simulink model "HESS_VBWF"  (R2023a)
settings: Solver=FixedStepAuto  StartTime=0.0  StopTime=2.5  RelTol=1e-3
undefined symbols (not defined in the file): Acid, BE, Lead, ode23tb, trap, Ts
libraries: spsMosfetLib x5, spsSeriesRLCBranchLib x5, slpidlib x3, spsCurrentMeasurementLib x3, spsPWMGeneratorDCDCLib x2, spsMeanLib x2, rfmathmodels2 x1, spsBatteryLib x1, spsVoltageMeasurementLib x1, spsPVArrayLib x1, spsDiodeLib x1, spsSupercapacitorLib x1
settings Model: Creator=bomma  LastModifiedBy=bomma

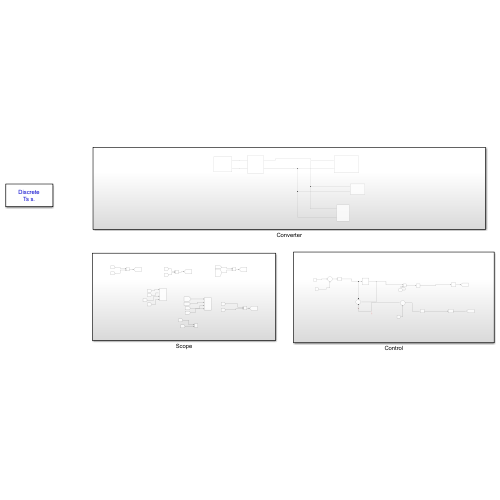
[thumbnail: Simulink's stored preview of the top-level diagram]
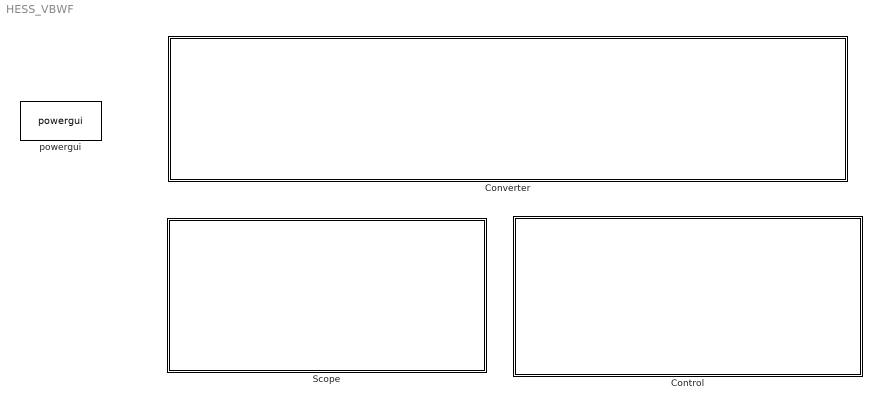
== system HESS_VBWF ==
  Control : Subsystem
  Converter : Subsystem
  Scope : Subsystem
  powergui : spspowerguiLib/powergui  Priority=1  SimulationMode=Discrete  SampleTime=Ts  frequency=60  Iterations=50  frequencyindice=0  Pbase=100e6  ErrMax=1e-4  UnitsV=kV  UnitsW=MW  buscounter=0  FunctionMessages=off  echomessages=off  EnableUseOfTLC=off  CurrentSourceSwitches=off  DisableSnubberDevices=off  DisableRonSwitches=off  DisableVfSwitches=off  DisplayEquations=off  AutomaticDiscreteSolvers=off  SolverType=Tustin/Backward Euler (TBE)  Interpol=off  ExternalGateDelay=off  methode=off  Ts=100  x0status=blocks  SPID=on  SwTol=0  HookPort=off  NonlinearTolerance=1e-4  nMaxIteration=100  ContinueOnMaxIteration=off  RestoreLinks=warning  ResistiveCurrentMeasurement=off  Frange=[0:2:500]  Ylog=off  Xlog=on  ShowGrid=off  save=off  variable=ZData  structure=0  ZoomFFT=off  StartTime=0.0  cycles=1  DisplayStyle=1  fundamental=60  FreqAxis=off  MaxFrequency=1000  frequencyindicesteady=1  RmsSteady=1  display=off

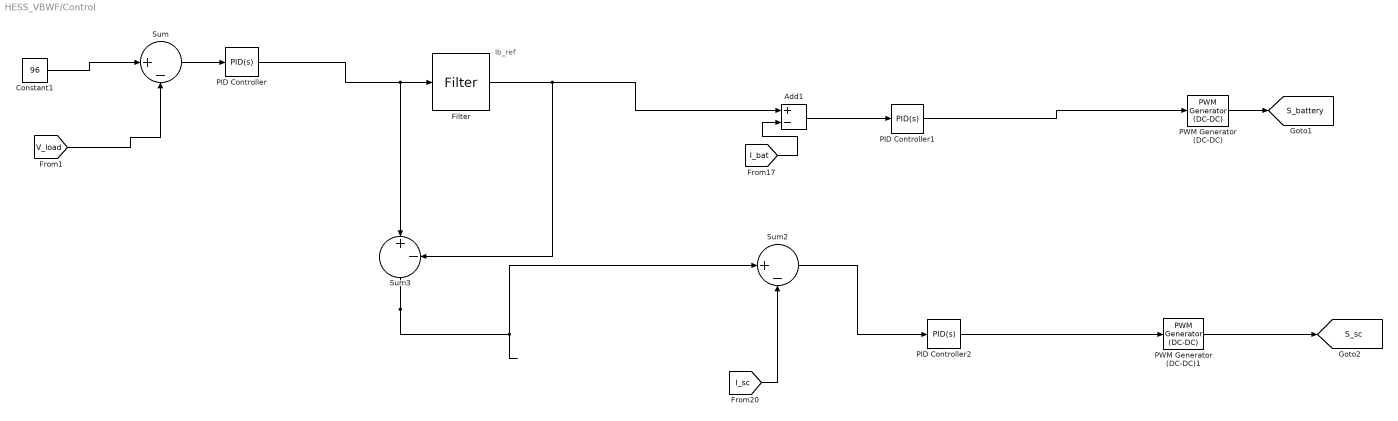
== system HESS_VBWF/Control ==
  note: Ib_ref
  Add1 : Sum  Inputs=+-
  Constant1 : Constant  Value=96
  Filter : rfmathmodels2/Filter  DesignMethod=Butterworth  ResponseType=Lowpass  UseFilterOrder=on  FilterOrder=3  PassFreq_lp=1e9  PassFreq_hp=2000000000  PassFreq_bp=[2000000000 3000000000]  PassFreq_bs=[1000000000 4000000000]  PassAtten=10*log10(2)  StopFreq_lp=2000000000  StopFreq_hp=1000000000  StopFreq_bp=[1500000000 3500000000]  StopFreq_bs=[2100000000 2900000000]  StopAtten=40  CarrierFrequency=1e9  SignalBandwidth=10000000  SimulateUsing=Interpreted execution  ModelingDomain=Time domain (Fixed step)  SolverFixedStep=NDF2  SolverODE=ode23tb (trap+BE)  PoleFitting=Share all poles  RationalArguments={ 'Tolerance', -40, 'TendsToZero', false, 'MaxPoles', 48, 'Qlimit', inf }  LengthFIR=128  PlotType1=S21  Plot1Units=Magnitude (dB)  Plot1ArgumentsImpulse=[1e-11 1e4]  Plot1ArgumentsStep=[1e-11 1e4 1e-10]  PlotType2=None  Plot2Units=Magnitude (dB)  Plot2ArgumentsImpulse=[1e-11 1e4]  Plot2ArgumentsStep=[1e-11 1e4 1e-10]  FrequencyPoints=logspace(8,10,2001)  XaxisScale=Linear  YaxisScale=Linear
  PID Controller : slpidlib/PID Controller  Controller=PID  Form=Parallel  TimeDomain=Continuous-time  UseExternalTs=off  SampleTime=-1  IntegratorMethod=Forward Euler  FilterMethod=Forward Euler  ControllerParametersSource=internal  P=1  I=1  UseKiTs=off  D=0  N=100  UseFilter=on  TunerSelectOption=Transfer Function Based (PID Tuner App)  InitialConditionSource=internal  InitialConditionForIntegrator=0  InitialConditionForFilter=0  DifferentiatorICPrevScaledInput=0  ExternalReset=none  TrackingMode=off  Kt=1  LimitOutput=off  SatLimitsSource=internal  UpperSaturationLimit=inf  LowerSaturationLimit=-inf  LinearizeAsGain=on  AntiWindupMode=none  Kb=1  LimitIntegrator=off  UpperIntegratorSaturationLimit=inf  LowerIntegratorSaturationLimit=-inf  POutMin=[]  POutMax=[]  IOutMin=[]  IOutMax=[]  DOutMin=[]  DOutMax=[]  NOutMin=[]  NOutMax=[]  SumOutMin=[]  SumOutMax=[]  SaturationOutMin=[]  SaturationOutMax=[]  PParamMin=[]  PParamMax=[]  IParamMin=[]  IParamMax=[]  DParamMin=[]  DParamMax=[]  NParamMin=[]  NParamMax=[]  KbParamMin=[]  KbParamMax=[]  KtParamMin=[]  KtParamMax=[]  KbOutMin=[]  KbOutMax=[]  KtOutMin=[]  KtOutMax=[]  IntegratorOutMin=[]  IntegratorOutMax=[]  FilterOutMin=[]  FilterOutMax=[]  SumI1OutMin=[]  SumI1OutMax=[]  SumI2OutMin=[]  SumI2OutMax=[]  SumI3OutMin=[]  SumI3OutMax=[]  SumI4OutMin=[]  SumI4OutMax=[]  SumDOutMin=[]  SumDOutMax=[]  DifferentiatorOutMin=[]  DifferentiatorOutMax=[]  FilterDiffOutCoefMin=[]  FilterDiffOutCoefMax=[]  ReciprocalOutMin=[]  ReciprocalOutMax=[]  SumDenOutMin=[]  SumDenOutMax=[]  SumNumOutMin=[]  SumNumOutMax=[]  DivideOutMin=[]  DivideOutMax=[]  UdiffTsProdOutMin=[]  UdiffTsProdOutMax=[]  NTsProdOutMin=[]  NTsProdOutMax=[]  UintegralTsProdOutMin=[]  UintegralTsProdOutMax=[]  UngainTsProdOutMin=[]  UngainTsProdOutMax=[]  ClampingZeroOutDataTypeStr=Inherit: Inherit via back propagation  ClampingZeroOutMin=[]  ClampingZeroOutMax=[]  FilterDenConstantOutDataTypeStr=Inherit: Inherit via back propagation  FilterDenConstantOutMin=[]  FilterDenConstantOutMax=[]  PCopyOutDataTypeStr=Inherit: Inherit via back propagation  PCopyOutMin=[]  PCopyOutMax=[]  NCopyOutDataTypeStr=Inherit: Inherit via back propagation  NCopyOutMin=[]  NCopyOutMax=[]  IntegratorContinuousStateAttributes=''  IntegratorStateMustResolveToSignalObject=off  IntegratorRTWStateStorageClass=Auto  FilterContinuousStateAttributes=''  FilterStateMustResolveToSignalObject=off  FilterRTWStateStorageClass=Auto  ParallelPVariant=InternalParameters  IdealPVariant=Disabled  IVariant=InternalParameters  DVariant=InternalParameters  IntegratorVariant=Continuous  SatVariant=Disabled  AWVariant=Passthrough  PCopyVariant=Disabled  TRVariant=Disabled  FdbkBlocksVariant=Forward  IdealPFdbkVariant=Disabled  SatFdbkVariant=Disabled  DerivativeFilterVariant=ContFilter  NVariant=InternalParameters  NCopyVariant=Disabled  FilterICVariant=InternalICsFilter  IntegratorICVariant=InternalICs  ExternalResetVariant=Disabled  TRSumVariant=Passthrough  SumFdbkVariant=Disabled  SumVariant=Sum_PID  TsampFilterVariant=InternalTs  TsampNgainVariant=Passthrough  TsampIntegralVariant=Passthrough  ExternalSaturationOutDataTypeStr=Inherit: Same as second input
  PID Controller1 : slpidlib/PID Controller  Controller=PID  Form=Parallel  TimeDomain=Continuous-time  UseExternalTs=off  SampleTime=-1  IntegratorMethod=Forward Euler  FilterMethod=Forward Euler  ControllerParametersSource=internal  P=1  I=1  UseKiTs=off  D=0  N=100  UseFilter=on  TunerSelectOption=Transfer Function Based (PID Tuner App)  InitialConditionSource=internal  InitialConditionForIntegrator=0  InitialConditionForFilter=0  DifferentiatorICPrevScaledInput=0  ExternalReset=none  TrackingMode=off  Kt=1  LimitOutput=off  SatLimitsSource=internal  UpperSaturationLimit=inf  LowerSaturationLimit=-inf  LinearizeAsGain=on  AntiWindupMode=none  Kb=1  LimitIntegrator=off  UpperIntegratorSaturationLimit=inf  LowerIntegratorSaturationLimit=-inf  POutMin=[]  POutMax=[]  IOutMin=[]  IOutMax=[]  DOutMin=[]  DOutMax=[]  NOutMin=[]  NOutMax=[]  SumOutMin=[]  SumOutMax=[]  SaturationOutMin=[]  SaturationOutMax=[]  PParamMin=[]  PParamMax=[]  IParamMin=[]  IParamMax=[]  DParamMin=[]  DParamMax=[]  NParamMin=[]  NParamMax=[]  KbParamMin=[]  KbParamMax=[]  KtParamMin=[]  KtParamMax=[]  KbOutMin=[]  KbOutMax=[]  KtOutMin=[]  KtOutMax=[]  IntegratorOutMin=[]  IntegratorOutMax=[]  FilterOutMin=[]  FilterOutMax=[]  SumI1OutMin=[]  SumI1OutMax=[]  SumI2OutMin=[]  SumI2OutMax=[]  SumI3OutMin=[]  SumI3OutMax=[]  SumI4OutMin=[]  SumI4OutMax=[]  SumDOutMin=[]  SumDOutMax=[]  DifferentiatorOutMin=[]  DifferentiatorOutMax=[]  FilterDiffOutCoefMin=[]  FilterDiffOutCoefMax=[]  ReciprocalOutMin=[]  ReciprocalOutMax=[]  SumDenOutMin=[]  SumDenOutMax=[]  SumNumOutMin=[]  SumNumOutMax=[]  DivideOutMin=[]  DivideOutMax=[]  UdiffTsProdOutMin=[]  UdiffTsProdOutMax=[]  NTsProdOutMin=[]  NTsProdOutMax=[]  UintegralTsProdOutMin=[]  UintegralTsProdOutMax=[]  UngainTsProdOutMin=[]  UngainTsProdOutMax=[]  ClampingZeroOutDataTypeStr=Inherit: Inherit via back propagation  ClampingZeroOutMin=[]  ClampingZeroOutMax=[]  FilterDenConstantOutDataTypeStr=Inherit: Inherit via back propagation  FilterDenConstantOutMin=[]  FilterDenConstantOutMax=[]  PCopyOutDataTypeStr=Inherit: Inherit via back propagation  PCopyOutMin=[]  PCopyOutMax=[]  NCopyOutDataTypeStr=Inherit: Inherit via back propagation  NCopyOutMin=[]  NCopyOutMax=[]  IntegratorContinuousStateAttributes=''  IntegratorStateMustResolveToSignalObject=off  IntegratorRTWStateStorageClass=Auto  FilterContinuousStateAttributes=''  FilterStateMustResolveToSignalObject=off  FilterRTWStateStorageClass=Auto  ParallelPVariant=InternalParameters  IdealPVariant=Disabled  IVariant=InternalParameters  DVariant=InternalParameters  IntegratorVariant=Continuous  SatVariant=Disabled  AWVariant=Passthrough  PCopyVariant=Disabled  TRVariant=Disabled  FdbkBlocksVariant=Forward  IdealPFdbkVariant=Disabled  SatFdbkVariant=Disabled  DerivativeFilterVariant=ContFilter  NVariant=InternalParameters  NCopyVariant=Disabled  FilterICVariant=InternalICsFilter  IntegratorICVariant=InternalICs  ExternalResetVariant=Disabled  TRSumVariant=Passthrough  SumFdbkVariant=Disabled  SumVariant=Sum_PID  TsampFilterVariant=InternalTs  TsampNgainVariant=Passthrough  TsampIntegralVariant=Passthrough  ExternalSaturationOutDataTypeStr=Inherit: Same as second input
  PID Controller2 : slpidlib/PID Controller  Controller=PID  Form=Parallel  TimeDomain=Continuous-time  UseExternalTs=off  SampleTime=-1  IntegratorMethod=Forward Euler  FilterMethod=Forward Euler  ControllerParametersSource=internal  P=1  I=1  UseKiTs=off  D=0  N=100  UseFilter=on  TunerSelectOption=Transfer Function Based (PID Tuner App)  InitialConditionSource=internal  InitialConditionForIntegrator=0  InitialConditionForFilter=0  DifferentiatorICPrevScaledInput=0  ExternalReset=none  TrackingMode=off  Kt=1  LimitOutput=off  SatLimitsSource=internal  UpperSaturationLimit=inf  LowerSaturationLimit=-inf  LinearizeAsGain=on  AntiWindupMode=none  Kb=1  LimitIntegrator=off  UpperIntegratorSaturationLimit=inf  LowerIntegratorSaturationLimit=-inf  POutMin=[]  POutMax=[]  IOutMin=[]  IOutMax=[]  DOutMin=[]  DOutMax=[]  NOutMin=[]  NOutMax=[]  SumOutMin=[]  SumOutMax=[]  SaturationOutMin=[]  SaturationOutMax=[]  PParamMin=[]  PParamMax=[]  IParamMin=[]  IParamMax=[]  DParamMin=[]  DParamMax=[]  NParamMin=[]  NParamMax=[]  KbParamMin=[]  KbParamMax=[]  KtParamMin=[]  KtParamMax=[]  KbOutMin=[]  KbOutMax=[]  KtOutMin=[]  KtOutMax=[]  IntegratorOutMin=[]  IntegratorOutMax=[]  FilterOutMin=[]  FilterOutMax=[]  SumI1OutMin=[]  SumI1OutMax=[]  SumI2OutMin=[]  SumI2OutMax=[]  SumI3OutMin=[]  SumI3OutMax=[]  SumI4OutMin=[]  SumI4OutMax=[]  SumDOutMin=[]  SumDOutMax=[]  DifferentiatorOutMin=[]  DifferentiatorOutMax=[]  FilterDiffOutCoefMin=[]  FilterDiffOutCoefMax=[]  ReciprocalOutMin=[]  ReciprocalOutMax=[]  SumDenOutMin=[]  SumDenOutMax=[]  SumNumOutMin=[]  SumNumOutMax=[]  DivideOutMin=[]  DivideOutMax=[]  UdiffTsProdOutMin=[]  UdiffTsProdOutMax=[]  NTsProdOutMin=[]  NTsProdOutMax=[]  UintegralTsProdOutMin=[]  UintegralTsProdOutMax=[]  UngainTsProdOutMin=[]  UngainTsProdOutMax=[]  ClampingZeroOutDataTypeStr=Inherit: Inherit via back propagation  ClampingZeroOutMin=[]  ClampingZeroOutMax=[]  FilterDenConstantOutDataTypeStr=Inherit: Inherit via back propagation  FilterDenConstantOutMin=[]  FilterDenConstantOutMax=[]  PCopyOutDataTypeStr=Inherit: Inherit via back propagation  PCopyOutMin=[]  PCopyOutMax=[]  NCopyOutDataTypeStr=Inherit: Inherit via back propagation  NCopyOutMin=[]  NCopyOutMax=[]  IntegratorContinuousStateAttributes=''  IntegratorStateMustResolveToSignalObject=off  IntegratorRTWStateStorageClass=Auto  FilterContinuousStateAttributes=''  FilterStateMustResolveToSignalObject=off  FilterRTWStateStorageClass=Auto  ParallelPVariant=InternalParameters  IdealPVariant=Disabled  IVariant=InternalParameters  DVariant=InternalParameters  IntegratorVariant=Continuous  SatVariant=Disabled  AWVariant=Passthrough  PCopyVariant=Disabled  TRVariant=Disabled  FdbkBlocksVariant=Forward  IdealPFdbkVariant=Disabled  SatFdbkVariant=Disabled  DerivativeFilterVariant=ContFilter  NVariant=InternalParameters  NCopyVariant=Disabled  FilterICVariant=InternalICsFilter  IntegratorICVariant=InternalICs  ExternalResetVariant=Disabled  TRSumVariant=Passthrough  SumFdbkVariant=Disabled  SumVariant=Sum_PID  TsampFilterVariant=InternalTs  TsampNgainVariant=Passthrough  TsampIntegralVariant=Passthrough  ExternalSaturationOutDataTypeStr=Inherit: Same as second input
  PWM Generator (DC-DC) : spsPWMGeneratorDCDCLib/PWM Generator (DC-DC)  Fsw=10e3  Ts=0
  PWM Generator (DC-DC)1 : spsPWMGeneratorDCDCLib/PWM Generator (DC-DC)  Fsw=10e3  Ts=0
  Sum : Sum  Inputs=|+-
  Sum2 : Sum  Inputs=|+-
  Sum3 : Sum  Inputs=|+-
  tag scope: S_battery=global, S_sc=global
  wires:
  Sum3/1 -> Sum2/1
  [V_load] -> Sum/2
  Constant1/1 -> Sum/1
  PWM Generator (DC-DC)/1 -> [S_battery]
  [I_bat] -> Add1/2
  [I_sc] -> Sum2/2
  Filter/1 -> Sum3/2, Add1/1
  Sum/1 -> PID Controller/1
  PID Controller/1 -> Sum3/1, Filter/1
  Add1/1 -> PID Controller1/1
  PID Controller1/1 -> PWM Generator (DC-DC)/1
  PID Controller2/1 -> PWM Generator (DC-DC)1/1
  Sum2/1 -> PID Controller2/1
  PWM Generator (DC-DC)1/1 -> [S_sc]

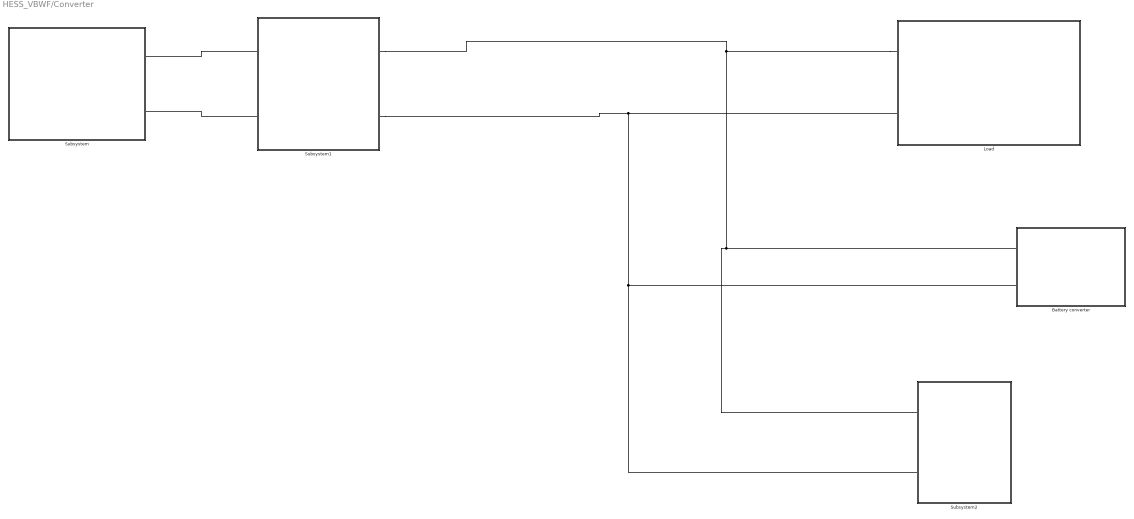
== system HESS_VBWF/Converter ==
  Battery converter : Subsystem
  Load : Subsystem
  Subsystem : Subsystem
  Subsystem1 : Subsystem
  Subsystem2 : Subsystem
  connections:
  Subsystem1/LConn1 -- Subsystem/RConn1
  Subsystem1/LConn2 -- Subsystem/RConn2
  Subsystem1/RConn2 -- Subsystem2/LConn2 -- Battery converter/LConn2 -- Load/LConn2
  Load/LConn1 -- Subsystem1/RConn1 -- Subsystem2/LConn1 -- Battery converter/LConn1

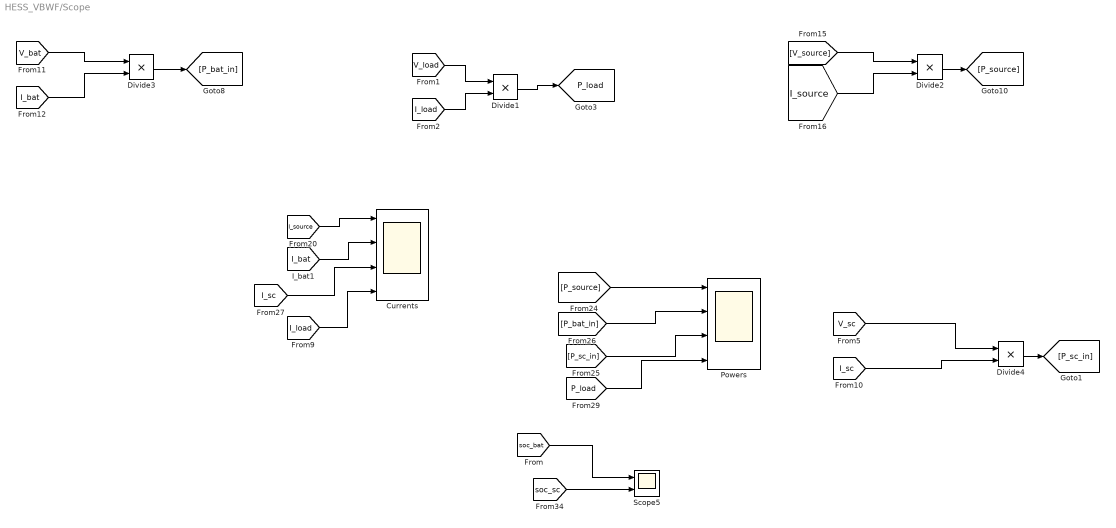
== system HESS_VBWF/Scope ==
  Currents : Scope  NumInputPorts=4
  Divide{1..4} (4 alike) : Product  Inputs=**
  Powers : Scope  NumInputPorts=4
  Scope5 : Scope  NumInputPorts=2
  tag scope: P_load=global
  wires:
  [V_bat] -> Divide3/1
  [I_bat] -> Divide3/2
  [I_bat] -> Currents/2
  Divide3/1 -> [P_bat_in]
  [V_source] -> Divide2/1
  [P_sc_in] -> Powers/3
  [P_bat_in] -> Powers/2
  [I_load] -> Divide1/2
  [I_source] -> Divide2/2
  Divide2/1 -> [P_source]
  [V_load] -> Divide1/1
  Divide1/1 -> [P_load]
  [P_source] -> Powers/1
  [I_source] -> Currents/1
  Divide4/1 -> [P_sc_in]
  [V_sc] -> Divide4/1
  [I_sc] -> Divide4/2
  [I_load] -> Currents/4
  [I_sc] -> Currents/3
  [P_load] -> Powers/4
  [soc_bat] -> Scope5/1
  [soc_sc] -> Scope5/2

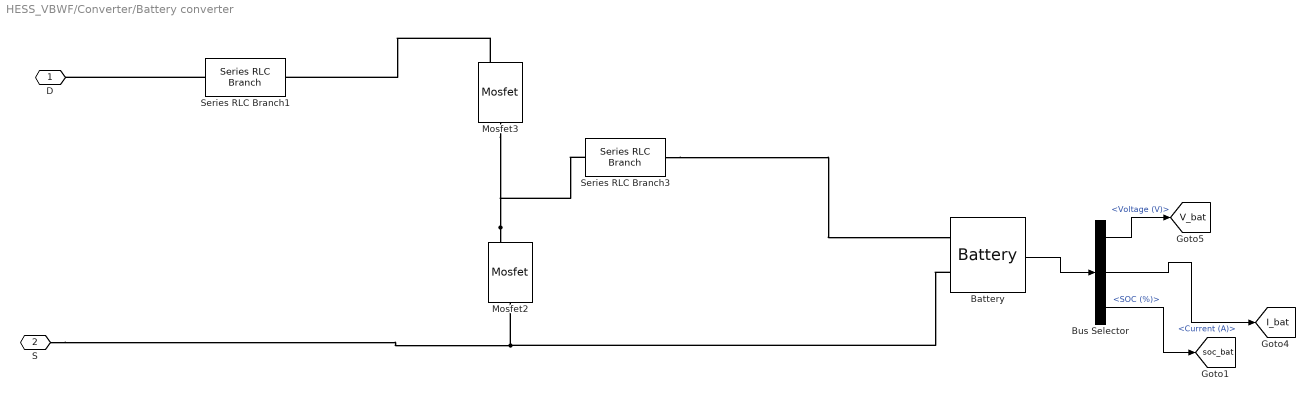
== system HESS_VBWF/Converter/Battery converter ==
  Battery : spsBatteryLib/Battery  BatType=Lead-Acid  ShowTempParam=off  ThermalPreset=no  ShowAgeParam=off  NomV=48  NomQ=28  SOC=79.997  Batt_Tr=10  PresetModel=on  MaxQ=29.1667  MinV=36  FullV=52.2632  Dis_rate=5.6  R=0.017143  Normal_OP=8.6878  expZone="[48.8684    0.0933333]"  current=[6.5 13 32.5]  Units=Time  Tci=20  NomT=20  T2=-30  MaxQ2=4.8  FullV2=7.1  Normal_OP2=5.655  expZone2="[6.58           1]"  Rca=0.6  ti=2000  Dp=0  Neq0=0  Tsim=1e6  Ta1=25  Qeol=5.4*0.9  Reol=0.013333*1.2  Char_age=[2.3478, 3]  Dis_age=[2.3478, 10]  N1=1500  N2=10500  N3=1000  N4=1400  Ta2=45  N5=950
  Bus Selector : BusSelector  OutputSignals=Voltage (V),Current (A),SOC (%)
  Mosfet2 : spsMosfetLib/Mosfet  Ron=0.1  Lon=0  Rd=0.01  Vfd=0  IC=0  Rs=1e5  Cs=inf  Measurements=off
  Mosfet3 : spsMosfetLib/Mosfet  Ron=0.1  Lon=0  Rd=0.01  Vfd=0  IC=0  Rs=1e5  Cs=inf  Measurements=off
  Series RLC Branch1 : spsSeriesRLCBranchLib/Series RLC Branch  LConnTagsString=__new0  RConnTagsString=__new0  BranchType=R  Resistance=0.01  Inductance=0.75e-3  SetiL0=off  InitialCurrent=0  Capacitance=1e-6  Setx0=off  InitialVoltage=0  Measurements=None
  Series RLC Branch3 : spsSeriesRLCBranchLib/Series RLC Branch  LConnTagsString=__new0  RConnTagsString=__new0  BranchType=L  Resistance=0.01  Inductance=2.3e-3  SetiL0=off  InitialCurrent=0  Capacitance=1e-6  Setx0=off  InitialVoltage=0  Measurements=None
  D : PMIOPort  Side=Left
  S : PMIOPort  Port=2  Side=Left
  tag scope: I_bat=global, V_bat=global, soc_bat=global
  wires:
  Bus Selector/2 -> [I_bat]  "<Current (A)>"
  Bus Selector/1 -> [V_bat]  "<Voltage (V)>"
  Battery/1 -> Bus Selector/1
  Bus Selector/3 -> [soc_bat]  "<SOC (%)>"
  connections:
  Series RLC Branch3/RConn1 -- Battery/LConn1
  Battery/LConn2 -- S/RConn1 -- Mosfet2/RConn1
  Mosfet2/LConn1 -- Series RLC Branch3/LConn1 -- Mosfet3/RConn1
  Series RLC Branch1/LConn1 -- D/RConn1
  Mosfet3/LConn1 -- Series RLC Branch1/RConn1

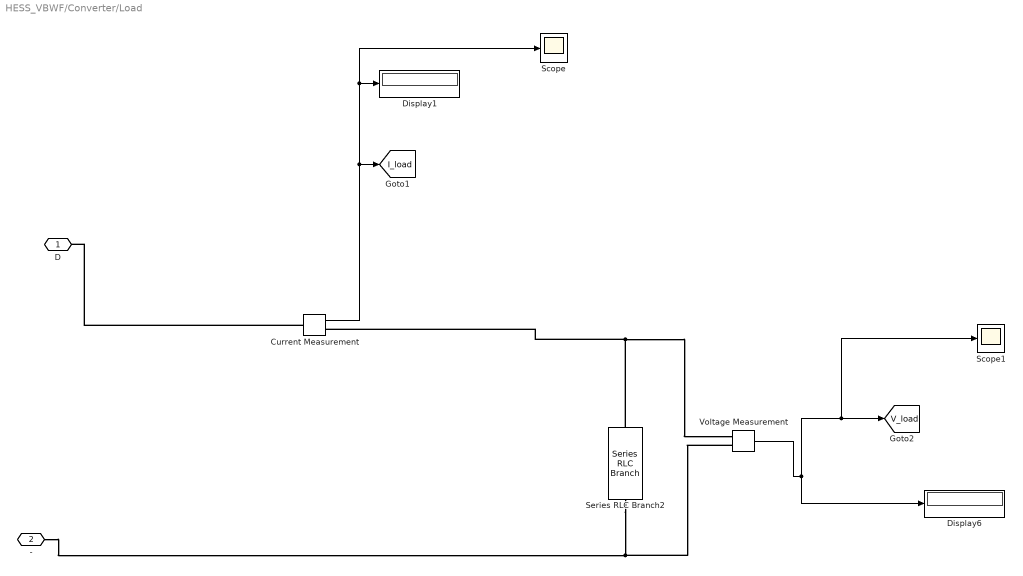
== system HESS_VBWF/Converter/Load ==
  Current Measurement : spsCurrentMeasurementLib/Current Measurement  PhasorSimulation=off  OutputType=Complex  PSBequivalent=0
  Display1 : Display
  Display6 : Display
  Scope : Scope
  Scope1 : Scope
  Series RLC Branch2 : spsSeriesRLCBranchLib/Series RLC Branch  LConnTagsString=__new0  RConnTagsString=__new0  BranchType=R  Resistance=48  Inductance=1e-3  SetiL0=off  InitialCurrent=0  Capacitance=1e-6  Setx0=off  InitialVoltage=0  Measurements=None
  Voltage Measurement : spsVoltageMeasurementLib/Voltage Measurement  PhasorSimulation=off  OutputType=Complex  PSBequivalent=0
  D : PMIOPort  Side=Left
  - : PMIOPort  Port=2  Side=Left
  tag scope: I_load=global, V_load=global
  wires:
  Voltage Measurement/1 -> Display6/1, Scope1/1, [V_load]
  Current Measurement/1 -> Scope/1, Display1/1, [I_load]
  connections:
  Current Measurement/RConn1 -- Series RLC Branch2/LConn1 -- Voltage Measurement/LConn1
  -/RConn1 -- Series RLC Branch2/RConn1 -- Voltage Measurement/LConn2
  Current Measurement/LConn1 -- D/RConn1

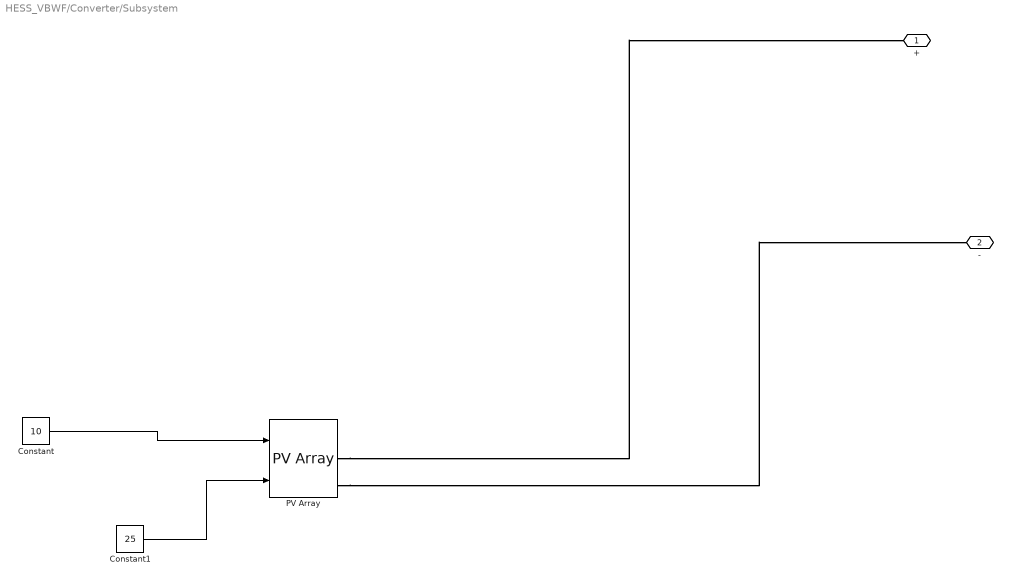
== system HESS_VBWF/Converter/Subsystem ==
  Constant : Constant  Value=10
  Constant1 : Constant  Value=25
  PV Array : spsPVArrayLib/PV Array  Npar=3  Nser=4  PlotType=one module @ 25 deg.C & specified irradiances  S_vec="[ 1000 800 500  250 ]"  Temp_C_vec="[0 25 50  ]"  ModuleName=Advance Power API-M310  PlotWhenSelected=on  Pm=310.284  Ncell=72  Voc=45  Isc=8.79  Vm=36.72  Im=8.45  beta_Voc_pc=-0.3244  alpha_Isc_pc=0.053322  beta_Voc=-0.14598  alpha_Isc=0.004687  IL=8.912  I0=8.1389e-11  nI=0.95714  Rsh=1483.2976  Rs=0.35123  RobustModel=off  RobustCellTemperature=313.3991  BAL=on  Tc=Tc  Tfilter=5e-5
  + : PMIOPort  Side=Right
  - : PMIOPort  Port=2  Side=Right
  wires:
  Constant/1 -> PV Array/1
  Constant1/1 -> PV Array/2
  connections:
  PV Array/RConn2 -- -/RConn1
  PV Array/RConn1 -- +/RConn1

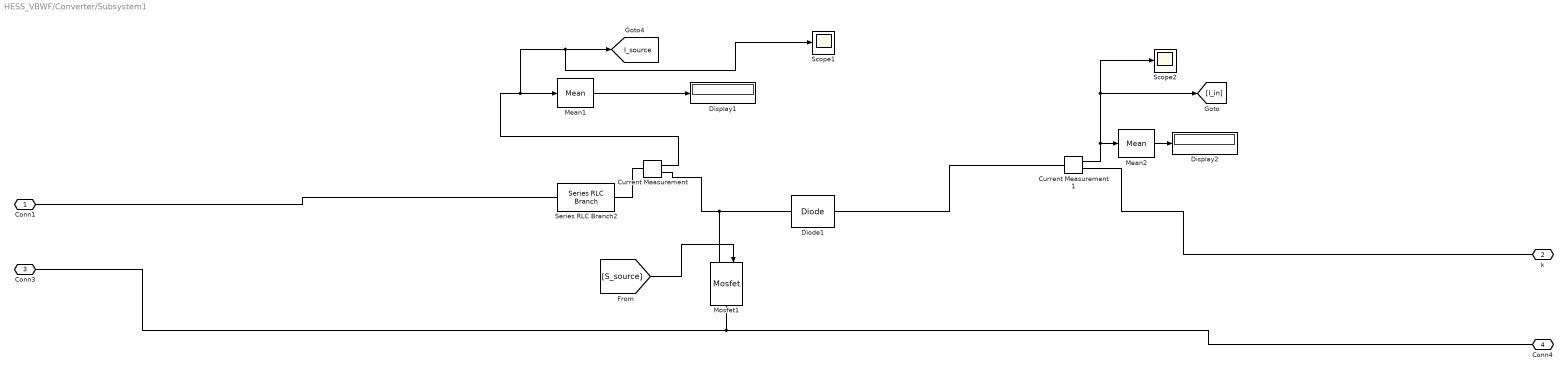
== system HESS_VBWF/Converter/Subsystem1 ==
  Current Measurement : spsCurrentMeasurementLib/Current Measurement  PhasorSimulation=off  OutputType=Complex  PSBequivalent=0
  Current Measurement1 : spsCurrentMeasurementLib/Current Measurement  PhasorSimulation=off  OutputType=Complex  PSBequivalent=0
  Diode1 : spsDiodeLib/Diode  Ron=0.001  Lon=0  Vf=0.8  IC=0  UseSnubber=0  Rs=500  Cs=250e-9  Measurements=off
  Display1 : Display
  Display2 : Display
  Mean1 : spsMeanLib/Mean  Freq=60  Vinit=0  Ts=0
  Mean2 : spsMeanLib/Mean  Freq=60  Vinit=0  Ts=0
  Mosfet1 : spsMosfetLib/Mosfet  Ron=0.1  Lon=0  Rd=0.01  Vfd=0  IC=0  Rs=1e5  Cs=inf  Measurements=off
  Scope1 : Scope
  Scope2 : Scope
  Series RLC Branch2 : spsSeriesRLCBranchLib/Series RLC Branch  LConnTagsString=__new0  RConnTagsString=__new0  BranchType=L  Resistance=0.1  Inductance=3.1e-3  SetiL0=off  InitialCurrent=0  Capacitance=10e-6  Setx0=off  InitialVoltage=0  Measurements=None
  Conn1 : PMIOPort  Side=Left
  k : PMIOPort  Port=2  Side=Right
  Conn3 : PMIOPort  Port=3  Side=Left
  Conn4 : PMIOPort  Port=4  Side=Right
  tag scope: I_source=global
  wires:
  Current Measurement/1 -> Scope1/1, [I_source], Mean1/1
  [S_source] -> Mosfet1/1
  Mean1/1 -> Display1/1
  Mean2/1 -> Display2/1
  Current Measurement1/1 -> Mean2/1, [I_in], Scope2/1
  connections:
  Current Measurement1/RConn1 -- k/RConn1
  Series RLC Branch2/LConn1 -- Conn1/RConn1
  Series RLC Branch2/RConn1 -- Current Measurement/LConn1
  Mosfet1/LConn1 -- Diode1/LConn1 -- Current Measurement/RConn1
  Conn3/RConn1 -- Conn4/RConn1 -- Mosfet1/RConn1
  Current Measurement1/LConn1 -- Diode1/RConn1

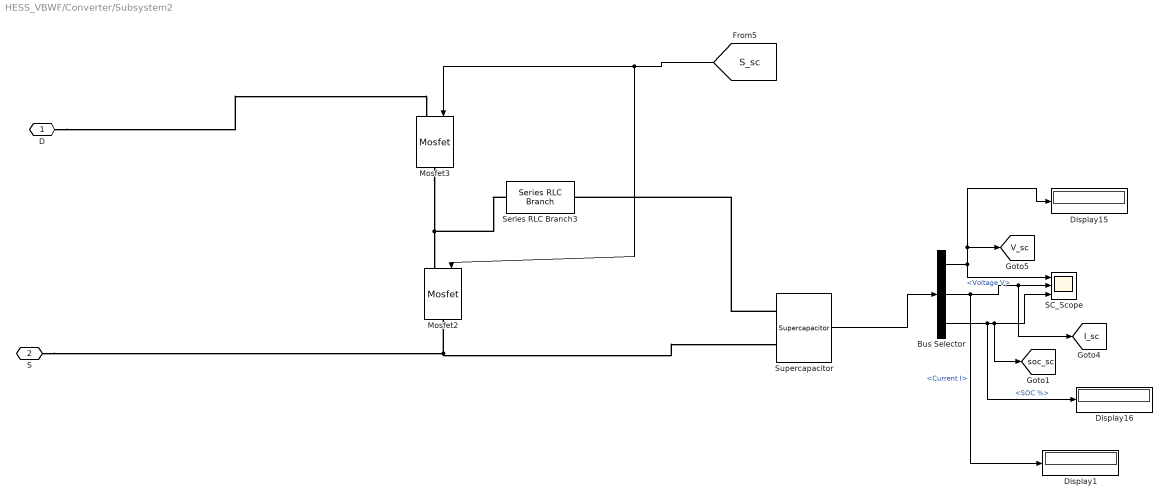
== system HESS_VBWF/Converter/Subsystem2 ==
  Bus Selector : BusSelector  OutputSignals=Voltage V,Current I,SOC %
  Display1 : Display
  Display15 : Display
  Display16 : Display
  Mosfet2 : spsMosfetLib/Mosfet  Ron=0.1  Lon=0  Rd=0.01  Vfd=0  IC=0  Rs=1e5  Cs=inf  Measurements=off
  Mosfet3 : spsMosfetLib/Mosfet  Ron=0.1  Lon=0  Rd=0.01  Vfd=0  IC=0  Rs=1e5  Cs=inf  Measurements=off
  SC_Scope : Scope  NumInputPorts=3
  Series RLC Branch3 : spsSeriesRLCBranchLib/Series RLC Branch  LConnTagsString=__new0  RConnTagsString=__new0  BranchType=L  Resistance=0.01  Inductance=2.3e-3  SetiL0=off  InitialCurrent=0  Capacitance=1e-6  Setx0=off  InitialVoltage=0  Measurements=None
  Supercapacitor : spsSupercapacitorLib/Supercapacitor  C=100  Rdc=8.9e-3  Voltage=48  Ns=1  Np=1  Vinit=48  Temp=38  PresetModel=off  EstParam=off  Nc=1  r=1e-9  epsilon=6.0208e-10  Ich=10  Vstern="[0.161  2.7  7.8]"  Self_dis=on  Ioc=10  Vself="[48  47.8  47.06  44.65]"  demandeplot=off  I="[10  20 100  500]"  Units=sec  Vmax=0  If=0  deltaV=0  alpha=0  sec=0
      settings: LibrarySourceBlock=sps_lib/Sources/Supercapacitor
  D : PMIOPort  Side=Left
  S : PMIOPort  Port=2  Side=Left
  tag scope: I_sc=global, V_sc=global, soc_sc=global
  wires:
  Supercapacitor/1 -> Bus Selector/1
  Bus Selector/2 -> Display1/1, [I_sc], SC_Scope/2  "<Current I>"
  Bus Selector/1 -> SC_Scope/1, Display15/1, [V_sc]  "<Voltage V>"
  Bus Selector/3 -> Display16/1, SC_Scope/3, [soc_sc]  "<SOC %>"
  [S_sc] -> Mosfet3/1, Mosfet2/1
  connections:
  Supercapacitor/LConn1 -- Series RLC Branch3/RConn1
  Mosfet3/RConn1 -- Mosfet2/LConn1 -- Series RLC Branch3/LConn1
  S/RConn1 -- Supercapacitor/LConn2 -- Mosfet2/RConn1
  D/RConn1 -- Mosfet3/LConn1
